simulink model "main"  (R2019b)
settings: Solver=FixedStepDiscrete  StartTime=0.0  StopTime=inf  RelTol=1e-3
undefined symbols (not defined in the file): jet, pause
libraries: simulink x3, dspvision x1, visionsources x1, visionanalysis x1
settings Model: Creator=fabote  LastModifiedBy=thema

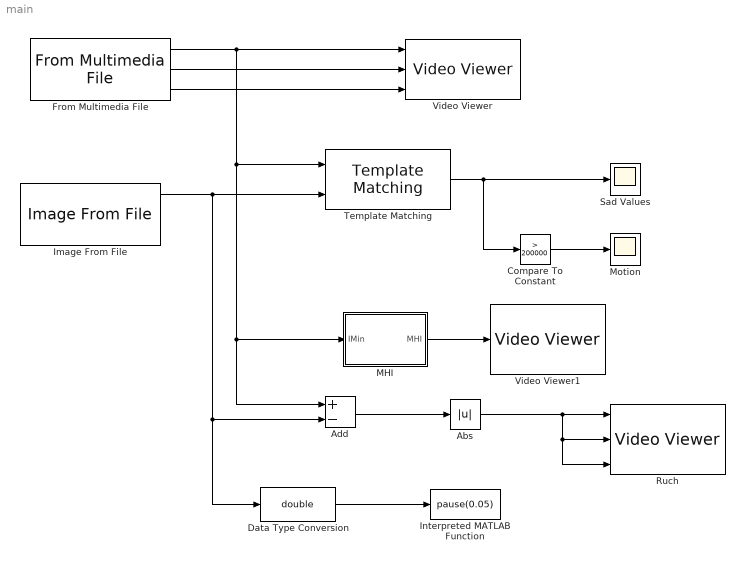
== system main ==
  Abs : Abs  OutDataTypeStr=uint8
  Add : Sum  Inputs=+-  OutDataTypeStr=int8  SaturateOnIntegerOverflow=on
  Compare To Constant : simulink/Logic and Bit Operations/Compare To Constant  relop=>  const=200000  OutDataTypeStr=boolean
  Data Type Conversion : DataTypeConversion  OutDataTypeStr=double
  From Multimedia File : dspvision/From Multimedia File  inputFilename=motion1.avi  readRange=[1 Inf]  loop=on  numPlays=inf  outputStreams=Video only  videoDataType=uint8  audioDataType=int16  inheritSampleTime=on  userDefinedSampleTime=1/30  noAudioOutput=off  isIntensityVideo=off  fourcc=RGB  colorVideoFormat=Separate color signals  outputEOF=off  dataOrg=Column-major  audioFrameSize=1024  computeAudioFrameSize=off  outSamplingMode=Sample based
      settings: SourceProductName=DSP System Toolbox  SourceProductBaseCode=DS
  Image From File : visionsources/Image From File  Tag=vipblks_nd  FileName=tlo0000.bmp  Ts=inf  imagePorts=Separate color signals  OutPortLabels=R|G|B  ImageDataType=Inherit from input image  sdImageDataType=uint(8)  Signed=on  WordLength=16  FractionLengthMode=User-defined  FractionLength=15
      settings: SourceProductName=Computer Vision Toolbox
  Interpreted MATLAB Function : MATLABFcn  MATLABFcn=pause(0.05)  OutputDimensions=0
  MHI : Subsystem  mask{tres=20, Tau=2}
      mask prompts: tres "Motion treshold"; Tau "Tau parameter"
  Motion : Scope
  Ruch : VideoViewer  imagePorts=separate color signals  FigPos=[887.4 725.2 257.6 179.2]
  "Sad Values " : Scope
  Template Matching : visionanalysis/Template Matching  metric=Sum of absolute differences  output=Metric matrix  method=Exhaustive  nMetric=off  nSize=3  roi=off  roiValid=off  roundingMode=Floor  overflowMode=off  prodOutputMode=Binary point scaling  prodOutputWordLength=32  prodOutputFracLength=0  prodOutputSlope=2^0  accumMode=Binary point scaling  accumWordLength=32  accumFracLength=0  accumSlope=2^0  outputMode=Binary point scaling  outputWordLength=32  outputFracLength=0  outputSlope=2^0
      settings: SourceProductName=Computer Vision Toolbox  SourceProductBaseCode=VP
  Video Viewer : VideoViewer  imagePorts=separate color signals  FigPos=[383.4 767.6 408 311.2]
  Video Viewer1 : VideoViewer  useColorMap=on  colormapValue=jet(2)  specRange=on  maxInputVal=2  FigPos=[1255.4 857.2 418.4 268.8]
  wires:
  From Multimedia File/1 -> Template Matching/1, MHI/1(IMin), Add/1, Video Viewer/1
  From Multimedia File/2 -> Video Viewer/2
  From Multimedia File/3 -> Video Viewer/3
  Image From File/1 -> Add/2, Data Type Conversion/1, Template Matching/2
  Template Matching/1 -> Compare To Constant/1, "Sad Values "/1
  Compare To Constant/1 -> Motion/1
  Data Type Conversion/1 -> Interpreted MATLAB Function/1
  Abs/1 -> Ruch/3, Ruch/2, Ruch/1
  Add/1 -> Abs/1
  MHI/1(MHI) -> Video Viewer1/1

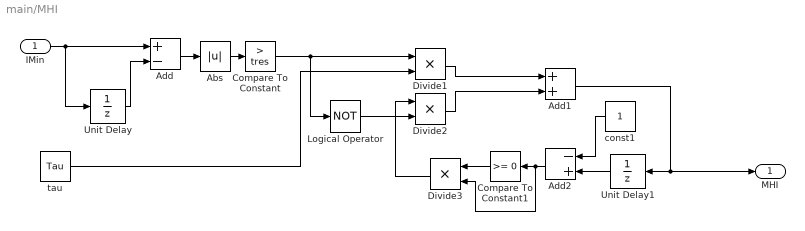
== system main/MHI ==
  IMin : Inport
  Abs : Abs
  Add : Sum  Inputs=+-  OutDataTypeStr=int16
  Add1 : Sum  OutDataTypeStr=double
  Add2 : Sum  Inputs=-+  OutDataTypeStr=double
  Compare To Constant : simulink/Logic and Bit Operations/Compare To Constant  relop=>  const=tres  OutDataTypeStr=uint8  ZeroCross=off
  Compare To Constant1 : simulink/Logic and Bit Operations/Compare To Constant  relop=>=  const=0  OutDataTypeStr=uint8  ZeroCross=off
  Divide1 : Product  Inputs=**
  Divide2 : Product  Inputs=**
  Divide3 : Product  Inputs=**
  Logical Operator : Logic  Operator=NOT  AllPortsSameDT=off  OutDataTypeStr=boolean
  Unit Delay : UnitDelay  SampleTime=-1  HasFrameUpgradeWarning=on
  Unit Delay1 : UnitDelay  SampleTime=-1  HasFrameUpgradeWarning=on
  const1 : Constant
  tau : Constant  Value=Tau
  MHI : Outport
  wires:
  Compare To Constant/1 -> Divide1/1, Logical Operator/1
  IMin/1 -> Unit Delay/1, Add/1
  Divide3/1 -> Divide2/1
  Compare To Constant1/1 -> Divide3/1
  Add2/1 -> Divide3/2, Compare To Constant1/1
  const1/1 -> Add2/1
  Unit Delay1/1 -> Add2/2
  Add1/1 -> MHI/1, Unit Delay1/1
  Divide2/1 -> Add1/2
  Divide1/1 -> Add1/1
  Logical Operator/1 -> Divide2/2
  tau/1 -> Divide1/2
  Abs/1 -> Compare To Constant/1
  Add/1 -> Abs/1
  Unit Delay/1 -> Add/2
